simulink library "MESSIN_Library"  (R2024a)
settings: Solver=VariableStepAuto  StartTime=0.0  StopTime=10.0  RelTol=1e-3
undefined symbols (not defined in the file or in its folder): actuatorCommand, commandedActuator, commandMode, externCommand, ready, remoteControlDevice, sensor, supervisor, timestampUTC, useXNAllocation
libraries: $bdroot x376, etargetslib x52, simulink x19
(part 3 of 5)

== system MESSIN_Library/State Message/Pack MESSIN State Message/Pack INS ==
  insLFK100 : Inport
  Bus Selector : BusSelector  OutputSignals=timestampUTC,latitude,longitude,heave,velocityNorth,velocityEast,velocityDown,roll,pitch,heading,bodyAngularRateX,bodyAngularRateY,bodyAngularRateZ,bodyAccelerationX,bodyAccelerationY,bodyAccelerationZ,details.mode,details.systemFailure,details.reducedAccuracy,details.statusWord1,details.statusWord2
  Byte Pack5 : etargetslib/Byte Pack  datatypes={'double','double','double','double','double','double','double','double','double','double','double','double','double','double','double','double','uint8','uint8','uint16','uint16'}  byteAlign=1
  Convert Double Network Byte Order{1..4,6..7,9..11,15,17..22} (16 alike) : $bdroot/Utilities/Convert Double Network Byte Order
  Convert Uint16 Network Byte Order : $bdroot/Utilities/Convert Uint16 Network Byte Order
  Convert Uint16 Network Byte Order1 : $bdroot/Utilities/Convert Uint16 Network Byte Order
  Data Type Conversion{1..4,6..7,10,12..13,15..19,21,63} (16 alike) : DataTypeConversion  OutDataTypeStr=double  SaturateOnIntegerOverflow=off  RndMeth=Floor
  Data Type Conversion22 : DataTypeConversion  OutDataTypeStr=uint8  SaturateOnIntegerOverflow=off  RndMeth=Floor
  Data Type Conversion23 : DataTypeConversion  OutDataTypeStr=uint16  SaturateOnIntegerOverflow=off  RndMeth=Floor
  Data Type Conversion24 : DataTypeConversion  OutDataTypeStr=uint16  SaturateOnIntegerOverflow=off  RndMeth=Floor
  Subsystem : Subsystem
  bytes : Outport
  wires:
  insLFK100/1 -> Bus Selector/1
  Byte Pack5/1 -> bytes/1
  Data Type Conversion63/1 -> Convert Double Network Byte Order9/1
  Bus Selector/1 -> Data Type Conversion63/1  "<timestampUTC>"
  Bus Selector/2 -> Data Type Conversion1/1  "<latitude>"
  Bus Selector/3 -> Data Type Conversion3/1  "<longitude>"
  Bus Selector/4 -> Data Type Conversion2/1  "<heave>"
  Bus Selector/5 -> Data Type Conversion7/1  "<velocityNorth>"
  Bus Selector/6 -> Data Type Conversion4/1  "<velocityEast>"
  Bus Selector/7 -> Data Type Conversion6/1  "<velocityDown>"
  Bus Selector/10 -> Data Type Conversion12/1  "<heading>"
  Bus Selector/9 -> Data Type Conversion10/1  "<pitch>"
  Bus Selector/8 -> Data Type Conversion13/1  "<roll>"
  Data Type Conversion1/1 -> Convert Double Network Byte Order1/1
  Data Type Conversion3/1 -> Convert Double Network Byte Order3/1
  Data Type Conversion2/1 -> Convert Double Network Byte Order2/1
  Data Type Conversion7/1 -> Convert Double Network Byte Order7/1
  Data Type Conversion4/1 -> Convert Double Network Byte Order4/1
  Data Type Conversion6/1 -> Convert Double Network Byte Order6/1
  Data Type Conversion13/1 -> Convert Double Network Byte Order11/1
  Data Type Conversion10/1 -> Convert Double Network Byte Order10/1
  Data Type Conversion12/1 -> Convert Double Network Byte Order15/1
  Data Type Conversion18/1 -> Convert Double Network Byte Order20/1
  Data Type Conversion19/1 -> Convert Double Network Byte Order21/1
  Data Type Conversion17/1 -> Convert Double Network Byte Order19/1
  Data Type Conversion21/1 -> Convert Double Network Byte Order22/1
  Data Type Conversion15/1 -> Convert Double Network Byte Order17/1
  Data Type Conversion16/1 -> Convert Double Network Byte Order18/1
  Bus Selector/16 -> Data Type Conversion18/1  "<bodyAccelerationZ>"
  Bus Selector/15 -> Data Type Conversion19/1  "<bodyAccelerationY>"
  Bus Selector/14 -> Data Type Conversion17/1  "<bodyAccelerationX>"
  Bus Selector/13 -> Data Type Conversion21/1  "<bodyAngularRateZ>"
  Bus Selector/12 -> Data Type Conversion15/1  "<bodyAngularRateY>"
  Bus Selector/11 -> Data Type Conversion16/1  "<bodyAngularRateX>"
  Bus Selector/17 -> Data Type Conversion22/1  "<mode>"
  Bus Selector/20 -> Data Type Conversion23/1  "<statusWord1>"
  Bus Selector/21 -> Data Type Conversion24/1  "<statusWord2>"
  Data Type Conversion23/1 -> Convert Uint16 Network Byte Order/1
  Data Type Conversion24/1 -> Convert Uint16 Network Byte Order1/1
  Bus Selector/18 -> Subsystem/1(bit0)  "<systemFailure>"
  Bus Selector/19 -> Subsystem/2(bit1)  "<reducedAccuracy>"
  Convert Double Network Byte Order20/1 -> Byte Pack5/16
  Convert Double Network Byte Order21/1 -> Byte Pack5/15
  Convert Double Network Byte Order19/1 -> Byte Pack5/14
  Convert Double Network Byte Order22/1 -> Byte Pack5/13
  Convert Double Network Byte Order17/1 -> Byte Pack5/12
  Convert Double Network Byte Order18/1 -> Byte Pack5/11
  Convert Double Network Byte Order15/1 -> Byte Pack5/10
  Convert Double Network Byte Order10/1 -> Byte Pack5/9
  Convert Double Network Byte Order11/1 -> Byte Pack5/8
  Convert Double Network Byte Order6/1 -> Byte Pack5/7
  Convert Double Network Byte Order4/1 -> Byte Pack5/6
  Convert Double Network Byte Order7/1 -> Byte Pack5/5
  Convert Double Network Byte Order2/1 -> Byte Pack5/4
  Convert Double Network Byte Order3/1 -> Byte Pack5/3
  Convert Double Network Byte Order1/1 -> Byte Pack5/2
  Convert Double Network Byte Order9/1 -> Byte Pack5/1
  Data Type Conversion22/1 -> Byte Pack5/17
  Subsystem/1(byte) -> Byte Pack5/18
  Convert Uint16 Network Byte Order1/1 -> Byte Pack5/20
  Convert Uint16 Network Byte Order/1 -> Byte Pack5/19

== system MESSIN_Library/State Message/Pack MESSIN State Message/Pack Info ==
  messinState : Inport
  Bus Selector1 : BusSelector  OutputSignals=timestampUTC
  Byte Pack : etargetslib/Byte Pack  datatypes={'double'}  byteAlign=1
  Convert Double Network Byte Order : $bdroot/Utilities/Convert Double Network Byte Order
  bytes : Outport
  wires:
  Bus Selector1/1 -> Convert Double Network Byte Order/1  "<timestampUTC>"
  Convert Double Network Byte Order/1 -> Byte Pack/1
  messinState/1 -> Bus Selector1/1
  Byte Pack/1 -> bytes/1

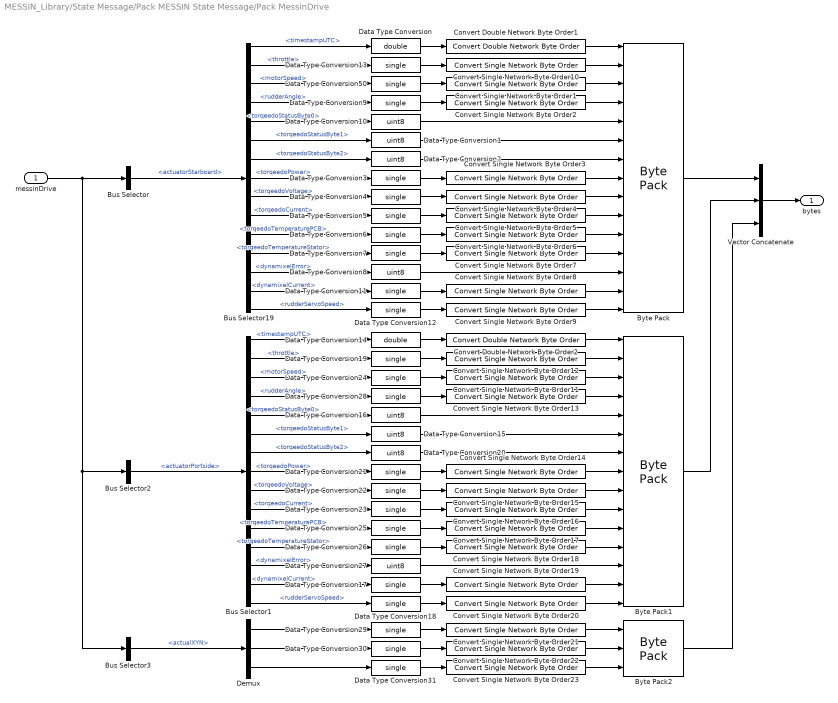
== system MESSIN_Library/State Message/Pack MESSIN State Message/Pack MessinDrive ==
  messinDrive : Inport
  Bus Selector : BusSelector  OutputSignals=actuatorStarboard
  Bus Selector1 : BusSelector  OutputSignals=timestampUTC,throttle,motorSpeed,rudderAngle,torqeedoStatusByte0,torqeedoStatusByte1,torqeedoStatusByte2,torqeedoPower,torqeedoVoltage,torqeedoCurrent,torqeedoTemperaturePCB,torqeedoTemperatureStator,dynamixelError,dynamixelCurrent,rudderServoSpeed
  Bus Selector19 : BusSelector  OutputSignals=timestampUTC,throttle,motorSpeed,rudderAngle,torqeedoStatusByte0,torqeedoStatusByte1,torqeedoStatusByte2,torqeedoPower,torqeedoVoltage,torqeedoCurrent,torqeedoTemperaturePCB,torqeedoTemperatureStator,dynamixelError,dynamixelCurrent,rudderServoSpeed
  Bus Selector2 : BusSelector  OutputSignals=actuatorPortside
  Bus Selector3 : BusSelector  OutputSignals=actualXYN
  Byte Pack : etargetslib/Byte Pack  datatypes={'double','single','single','single','uint8','uint8','uint8','single','single','single','single','single','uint8','single','single'}  byteAlign=1
  Byte Pack1 : etargetslib/Byte Pack  datatypes={'double','single','single','single','uint8','uint8','uint8','single','single','single','single','single','uint8','single','single'}  byteAlign=1
  Byte Pack2 : etargetslib/Byte Pack  datatypes={'single','single','single'}  byteAlign=1
  Convert Double Network Byte Order1 : $bdroot/Utilities/Convert Double Network Byte Order
  Convert Double Network Byte Order2 : $bdroot/Utilities/Convert Double Network Byte Order
  Convert Single Network Byte Order{1..23} (23 alike) : $bdroot/Utilities/Convert Single Network Byte Order
  Data Type Conversion : DataTypeConversion  OutDataTypeStr=double  SaturateOnIntegerOverflow=off  RndMeth=Floor
  Data Type Conversion{1..2,8,10,15..16,20,27} (8 alike) : DataTypeConversion  OutDataTypeStr=uint8  SaturateOnIntegerOverflow=off  RndMeth=Floor
  Data Type Conversion{3..7,9,11..13,17..19,21..26,28..31,50} (23 alike) : DataTypeConversion  OutDataTypeStr=single  SaturateOnIntegerOverflow=off  RndMeth=Floor
  Data Type Conversion14 : DataTypeConversion  OutDataTypeStr=double  SaturateOnIntegerOverflow=off  RndMeth=Floor
  Demux : Demux  Outputs=3
  Vector Concatenate : Concatenate  NumInputs=3
  bytes : Outport
  wires:
  Data Type Conversion/1 -> Convert Double Network Byte Order1/1
  Byte Pack/1 -> Vector Concatenate/1
  Vector Concatenate/1 -> bytes/1
  messinDrive/1 -> Bus Selector3/1, Bus Selector2/1, Bus Selector/1
  Bus Selector/1 -> Bus Selector19/1  "<actuatorStarboard>"
  Bus Selector19/1 -> Data Type Conversion/1  "<timestampUTC>"
  Bus Selector19/3 -> Data Type Conversion50/1  "<motorSpeed>"
  Data Type Conversion50/1 -> Convert Single Network Byte Order1/1
  Bus Selector19/4 -> Data Type Conversion9/1  "<rudderAngle>"
  Bus Selector19/5 -> Data Type Conversion10/1  "<torqeedoStatusByte0>"
  Data Type Conversion9/1 -> Convert Single Network Byte Order2/1
  Bus Selector19/6 -> Data Type Conversion1/1  "<torqeedoStatusByte1>"
  Bus Selector19/7 -> Data Type Conversion2/1  "<torqeedoStatusByte2>"
  Bus Selector19/8 -> Data Type Conversion3/1  "<torqeedoPower>"
  Bus Selector19/9 -> Data Type Conversion4/1  "<torqeedoVoltage>"
  Bus Selector19/10 -> Data Type Conversion5/1  "<torqeedoCurrent>"
  Bus Selector19/11 -> Data Type Conversion6/1  "<torqeedoTemperaturePCB>"
  Bus Selector19/12 -> Data Type Conversion7/1  "<torqeedoTemperatureStator>"
  Bus Selector19/13 -> Data Type Conversion8/1  "<dynamixelError>"
  Bus Selector19/14 -> Data Type Conversion11/1  "<dynamixelCurrent>"
  Bus Selector19/15 -> Data Type Conversion12/1  "<rudderServoSpeed>"
  Data Type Conversion3/1 -> Convert Single Network Byte Order3/1
  Data Type Conversion4/1 -> Convert Single Network Byte Order4/1
  Data Type Conversion5/1 -> Convert Single Network Byte Order5/1
  Data Type Conversion6/1 -> Convert Single Network Byte Order6/1
  Data Type Conversion7/1 -> Convert Single Network Byte Order7/1
  Data Type Conversion11/1 -> Convert Single Network Byte Order8/1
  Data Type Conversion12/1 -> Convert Single Network Byte Order9/1
  Data Type Conversion13/1 -> Convert Single Network Byte Order10/1
  Convert Double Network Byte Order1/1 -> Byte Pack/1
  Convert Single Network Byte Order10/1 -> Byte Pack/2
  Convert Single Network Byte Order1/1 -> Byte Pack/3
  Convert Single Network Byte Order2/1 -> Byte Pack/4
  Convert Single Network Byte Order3/1 -> Byte Pack/8
  Convert Single Network Byte Order4/1 -> Byte Pack/9
  Convert Single Network Byte Order5/1 -> Byte Pack/10
  Convert Single Network Byte Order6/1 -> Byte Pack/11
  Convert Single Network Byte Order7/1 -> Byte Pack/12
  Convert Single Network Byte Order8/1 -> Byte Pack/14
  Convert Single Network Byte Order9/1 -> Byte Pack/15
  Data Type Conversion10/1 -> Byte Pack/5
  Data Type Conversion1/1 -> Byte Pack/6
  Data Type Conversion2/1 -> Byte Pack/7
  Data Type Conversion8/1 -> Byte Pack/13
  Bus Selector19/2 -> Data Type Conversion13/1  "<throttle>"
  Bus Selector1/2 -> Data Type Conversion19/1  "<throttle>"
  Data Type Conversion27/1 -> Byte Pack1/13
  Data Type Conversion20/1 -> Byte Pack1/7
  Data Type Conversion15/1 -> Byte Pack1/6
  Data Type Conversion16/1 -> Byte Pack1/5
  Convert Single Network Byte Order20/1 -> Byte Pack1/15
  Convert Single Network Byte Order19/1 -> Byte Pack1/14
  Convert Single Network Byte Order18/1 -> Byte Pack1/12
  Convert Single Network Byte Order17/1 -> Byte Pack1/11
  Convert Single Network Byte Order16/1 -> Byte Pack1/10
  Convert Single Network Byte Order15/1 -> Byte Pack1/9
  Convert Single Network Byte Order14/1 -> Byte Pack1/8
  Convert Single Network Byte Order13/1 -> Byte Pack1/4
  Convert Single Network Byte Order11/1 -> Byte Pack1/3
  Convert Single Network Byte Order12/1 -> Byte Pack1/2
  Convert Double Network Byte Order2/1 -> Byte Pack1/1
  Data Type Conversion19/1 -> Convert Single Network Byte Order12/1
  Data Type Conversion18/1 -> Convert Single Network Byte Order20/1
  Data Type Conversion17/1 -> Convert Single Network Byte Order19/1
  Data Type Conversion26/1 -> Convert Single Network Byte Order18/1
  Data Type Conversion25/1 -> Convert Single Network Byte Order17/1
  Data Type Conversion23/1 -> Convert Single Network Byte Order16/1
  Data Type Conversion22/1 -> Convert Single Network Byte Order15/1
  Data Type Conversion21/1 -> Convert Single Network Byte Order14/1
  Bus Selector1/15 -> Data Type Conversion18/1  "<rudderServoSpeed>"
  Bus Selector1/14 -> Data Type Conversion17/1  "<dynamixelCurrent>"
  Bus Selector1/13 -> Data Type Conversion27/1  "<dynamixelError>"
  Bus Selector1/12 -> Data Type Conversion26/1  "<torqeedoTemperatureStator>"
  Bus Selector1/11 -> Data Type Conversion25/1  "<torqeedoTemperaturePCB>"
  Bus Selector1/10 -> Data Type Conversion23/1  "<torqeedoCurrent>"
  Bus Selector1/9 -> Data Type Conversion22/1  "<torqeedoVoltage>"
  Bus Selector1/8 -> Data Type Conversion21/1  "<torqeedoPower>"
  Bus Selector1/7 -> Data Type Conversion20/1  "<torqeedoStatusByte2>"
  Bus Selector1/6 -> Data Type Conversion15/1  "<torqeedoStatusByte1>"
  Data Type Conversion28/1 -> Convert Single Network Byte Order13/1
  Bus Selector1/5 -> Data Type Conversion16/1  "<torqeedoStatusByte0>"
  Bus Selector1/4 -> Data Type Conversion28/1  "<rudderAngle>"
  Data Type Conversion24/1 -> Convert Single Network Byte Order11/1
  Bus Selector1/3 -> Data Type Conversion24/1  "<motorSpeed>"
  Bus Selector1/1 -> Data Type Conversion14/1  "<timestampUTC>"
  Byte Pack1/1 -> Vector Concatenate/2
  Data Type Conversion14/1 -> Convert Double Network Byte Order2/1
  Bus Selector2/1 -> Bus Selector1/1  "<actuatorPortside>"
  Bus Selector3/1 -> Demux/1  "<actualXYN>"
  Demux/1 -> Data Type Conversion29/1
  Data Type Conversion29/1 -> Convert Single Network Byte Order21/1
  Data Type Conversion30/1 -> Convert Single Network Byte Order22/1
  Data Type Conversion31/1 -> Convert Single Network Byte Order23/1
  Demux/2 -> Data Type Conversion30/1
  Demux/3 -> Data Type Conversion31/1
  Convert Single Network Byte Order23/1 -> Byte Pack2/3
  Convert Single Network Byte Order22/1 -> Byte Pack2/2
  Convert Single Network Byte Order21/1 -> Byte Pack2/1
  Byte Pack2/1 -> Vector Concatenate/3

== system MESSIN_Library/State Message/Pack MESSIN State Message/Pack RCD ==
  rcd : Inport
  Bus Selector19 : BusSelector  OutputSignals=timestampUTC,joystickLeft,joystickRight
  Byte Pack : etargetslib/Byte Pack  datatypes={'double','single','single','single','single','single','single'}  byteAlign=1
  Convert Double Network Byte Order1 : $bdroot/Utilities/Convert Double Network Byte Order
  Convert Single Network Byte Order{1..6} (6 alike) : $bdroot/Utilities/Convert Single Network Byte Order
  Data Type Conversion : DataTypeConversion  OutDataTypeStr=double  SaturateOnIntegerOverflow=off  RndMeth=Floor
  Data Type Conversion{1..4,9,50} (6 alike) : DataTypeConversion  OutDataTypeStr=single  SaturateOnIntegerOverflow=off  RndMeth=Floor
  Demux : Demux  Outputs=3
  Demux1 : Demux  Outputs=3
  bytes : Outport
  wires:
  Data Type Conversion9/1 -> Convert Single Network Byte Order2/1
  Convert Single Network Byte Order2/1 -> Byte Pack/3
  Data Type Conversion50/1 -> Convert Single Network Byte Order1/1
  Bus Selector19/1 -> Data Type Conversion/1  "<timestampUTC>"
  rcd/1 -> Bus Selector19/1
  Convert Double Network Byte Order1/1 -> Byte Pack/1
  Data Type Conversion/1 -> Convert Double Network Byte Order1/1
  Convert Single Network Byte Order1/1 -> Byte Pack/2
  Byte Pack/1 -> bytes/1
  Data Type Conversion1/1 -> Convert Single Network Byte Order3/1
  Data Type Conversion2/1 -> Convert Single Network Byte Order6/1
  Data Type Conversion3/1 -> Convert Single Network Byte Order4/1
  Data Type Conversion4/1 -> Convert Single Network Byte Order5/1
  Demux/1 -> Data Type Conversion50/1
  Demux/2 -> Data Type Conversion9/1
  Demux/3 -> Data Type Conversion1/1
  Demux1/1 -> Data Type Conversion3/1
  Demux1/2 -> Data Type Conversion4/1
  Demux1/3 -> Data Type Conversion2/1
  Convert Single Network Byte Order3/1 -> Byte Pack/4
  Convert Single Network Byte Order4/1 -> Byte Pack/5
  Convert Single Network Byte Order5/1 -> Byte Pack/6
  Convert Single Network Byte Order6/1 -> Byte Pack/7
  Bus Selector19/2 -> Demux/1  "<joystickLeft>"
  Bus Selector19/3 -> Demux1/1  "<joystickRight>"

== system MESSIN_Library/State Message/Pack MESSIN State Message/Pack Supervisor ==
  supervisor : Inport
  Bus Selector1 : BusSelector  OutputSignals=internalOperationMode
  Bus Selector19 : BusSelector  OutputSignals=torqeedoPoweredOn,actuatorsEnabled,lightEnabled,actuatorsSynchronized,externModeEnabled
  Constant : Constant  Value=false  OutDataTypeStr=boolean
  Data Type Conversion : DataTypeConversion  OutDataTypeStr=uint8  SaturateOnIntegerOverflow=off  RndMeth=Floor
  Data Type Conversion1 : DataTypeConversion  OutDataTypeStr=uint8  SaturateOnIntegerOverflow=off  RndMeth=Floor
  Data Type Conversion2 : DataTypeConversion  OutDataTypeStr=boolean  SaturateOnIntegerOverflow=off  RndMeth=Floor
  Mux : Mux  Inputs=8
  Pack Bitfield : $bdroot/Utilities/Pack Bitfield
  Selector : Selector  InputPortWidth=8  IndexOptions=Index vector (dialog)  Indices=[8 7 6 5 4 3 2 1]  OutputSizes=1
  Vector Concatenate : Concatenate
  bytes : Outport
  wires:
  Vector Concatenate/1 -> bytes/1
  supervisor/1 -> Bus Selector1/1, Bus Selector19/1
  Bus Selector19/1 -> Mux/1  "<torqeedoPoweredOn>"
  Bus Selector19/2 -> Mux/2  "<actuatorsEnabled>"
  Bus Selector19/3 -> Mux/3  "<lightEnabled>"
  Bus Selector19/4 -> Mux/4  "<actuatorsSynchronized>"
  Bus Selector19/5 -> Mux/5  "<externModeEnabled>"
  Mux/1 -> Selector/1
  Constant/1 -> Mux/7, Mux/6, Mux/8
  Bus Selector1/1 -> Data Type Conversion1/1  "<internalOperationMode>"
  Pack Bitfield/1 -> Data Type Conversion/1
  Data Type Conversion/1 -> Vector Concatenate/1
  Data Type Conversion1/1 -> Vector Concatenate/2
  Selector/1 -> Data Type Conversion2/1
  Data Type Conversion2/1 -> Pack Bitfield/1

== system MESSIN_Library/State Message/Pack MESSIN State Message/Pack SystemDiagnostics ==
  systemDiagnostics : Inport
  Bus Selector1 : BusSelector  OutputSignals=details.hardware
  Bus Selector2 : BusSelector  OutputSignals=GNSS_OK,INS_OK,DVL_OK,ACTUATORS_OK,RCD_OK,EXTERN_OK
  Bus Selector3 : BusSelector  OutputSignals=details.network
  Bus Selector4 : BusSelector  OutputSignals=numTaskOverloads1,numTaskOverloads2,numTaskOverloads3,numCPUOverloads,numLostTicks,cpuTemperature
  Bus Selector5 : BusSelector  OutputSignals=internLinkUp,telemetryLinkUp,externLinkUp,internIncommingDataLFK100,internIncommingDataGNSSAsteRx3,internIncommingDataNortekDVL1000,internIncommingDataAirMAR,internIncommingDataBMS,internIncommingDataActuatorStarboard,internIncommingDataActuatorPortside,telemetryIncommingDataRCD,externIncommingData,firewallBlockedExternalInterface
  Bus Selector6 : BusSelector  OutputSignals=firewallAllowedExternalAddress
  Byte Pack : etargetslib/Byte Pack  datatypes={'uint32','uint32','uint32','uint32','uint32','single'}  byteAlign=1
  Byte Pack1 : etargetslib/Byte Pack  datatypes={'uint16','uint16','uint16','uint16','uint16'}  byteAlign=1
  Constant : Constant  Value=false  OutDataTypeStr=boolean
  Constant1 : Constant  Value=false  OutDataTypeStr=boolean
  Convert Single Network Byte Order : $bdroot/Utilities/Convert Single Network Byte Order
  Convert Uint16 Network Byte Order{,1..4} (5 alike) : $bdroot/Utilities/Convert Uint16 Network Byte Order
  Convert Uint32 Network Byte Order{,1..4} (5 alike) : $bdroot/Utilities/Convert Uint32 Network Byte Order
  Data Type Conversion{1..5} (5 alike) : DataTypeConversion  OutDataTypeStr=uint32  SaturateOnIntegerOverflow=off  RndMeth=Floor
  Data Type Conversion10 : DataTypeConversion  OutDataTypeStr=uint8  SaturateOnIntegerOverflow=off  RndMeth=Floor
  Data Type Conversion11 : DataTypeConversion  OutDataTypeStr=uint8  SaturateOnIntegerOverflow=off  RndMeth=Floor
  Data Type Conversion12 : DataTypeConversion  OutDataTypeStr=boolean  SaturateOnIntegerOverflow=off  RndMeth=Floor
  Data Type Conversion14 : DataTypeConversion  OutDataTypeStr=single  SaturateOnIntegerOverflow=off  RndMeth=Floor
  Data Type Conversion6 : DataTypeConversion  OutDataTypeStr=uint8  SaturateOnIntegerOverflow=off  RndMeth=Floor
  Data Type Conversion7 : DataTypeConversion  OutDataTypeStr=uint16  SaturateOnIntegerOverflow=off  RndMeth=Floor
  Data Type Conversion8 : DataTypeConversion  OutDataTypeStr=boolean  SaturateOnIntegerOverflow=off  RndMeth=Floor
  Data Type Conversion9 : DataTypeConversion  OutDataTypeStr=boolean  SaturateOnIntegerOverflow=off  RndMeth=Floor
  Demux : Demux  Outputs=5
  Mux : Mux  Inputs=8
  Mux1 : Mux  Inputs=8
  Mux2 : Mux  Inputs=8
  Pack Bitfield : $bdroot/Utilities/Pack Bitfield
  Pack Bitfield1 : $bdroot/Utilities/Pack Bitfield
  Pack Bitfield2 : $bdroot/Utilities/Pack Bitfield
  Selector : Selector  InputPortWidth=8  IndexOptions=Index vector (dialog)  Indices=[8 7 6 5 4 3 2 1]  OutputSizes=1
  Selector1 : Selector  InputPortWidth=8  IndexOptions=Index vector (dialog)  Indices=[8 7 6 5 4 3 2 1]  OutputSizes=1
  Selector2 : Selector  InputPortWidth=8  IndexOptions=Index vector (dialog)  Indices=[8 7 6 5 4 3 2 1]  OutputSizes=1
  Vector Concatenate : Concatenate  NumInputs=5
  bytes : Outport
  wires:
  systemDiagnostics/1 -> Bus Selector2/1, Bus Selector3/1, Bus Selector1/1
  Pack Bitfield/1 -> Data Type Conversion6/1
  Mux/1 -> Selector/1
  Constant/1 -> Mux/7, Mux/8
  Bus Selector1/1 -> Bus Selector4/1  "<hardware>"
  Bus Selector4/1 -> Data Type Conversion4/1  "<numTaskOverloads1>"
  Bus Selector4/2 -> Data Type Conversion1/1  "<numTaskOverloads2>"
  Bus Selector4/4 -> Data Type Conversion2/1  "<numCPUOverloads>"
  Bus Selector4/3 -> Data Type Conversion3/1  "<numTaskOverloads3>"
  Bus Selector4/5 -> Data Type Conversion5/1  "<numLostTicks>"
  Bus Selector3/1 -> Bus Selector6/1, Bus Selector5/1  "<network>"
  Constant1/1 -> Mux2/7, Mux2/6, Mux2/8
  Pack Bitfield1/1 -> Data Type Conversion10/1
  Mux1/1 -> Selector1/1
  Pack Bitfield2/1 -> Data Type Conversion11/1
  Mux2/1 -> Selector2/1
  Data Type Conversion4/1 -> Convert Uint32 Network Byte Order/1
  Data Type Conversion1/1 -> Convert Uint32 Network Byte Order1/1
  Data Type Conversion2/1 -> Convert Uint32 Network Byte Order3/1
  Data Type Conversion3/1 -> Convert Uint32 Network Byte Order2/1
  Data Type Conversion5/1 -> Convert Uint32 Network Byte Order4/1
  Byte Pack/1 -> Vector Concatenate/2
  Data Type Conversion6/1 -> Vector Concatenate/1
  Data Type Conversion10/1 -> Vector Concatenate/3
  Data Type Conversion11/1 -> Vector Concatenate/4
  Bus Selector6/1 -> Data Type Conversion7/1  "<firewallAllowedExternalAddress>"
  Data Type Conversion7/1 -> Demux/1
  Demux/1 -> Convert Uint16 Network Byte Order/1
  Demux/2 -> Convert Uint16 Network Byte Order1/1
  Demux/3 -> Convert Uint16 Network Byte Order2/1
  Demux/4 -> Convert Uint16 Network Byte Order3/1
  Demux/5 -> Convert Uint16 Network Byte Order4/1
  Byte Pack1/1 -> Vector Concatenate/5
  Vector Concatenate/1 -> bytes/1
  Selector/1 -> Data Type Conversion8/1
  Selector1/1 -> Data Type Conversion9/1
  Selector2/1 -> Data Type Conversion12/1
  Data Type Conversion8/1 -> Pack Bitfield/1
  Data Type Conversion9/1 -> Pack Bitfield1/1
  Data Type Conversion12/1 -> Pack Bitfield2/1
  Convert Uint16 Network Byte Order/1 -> Byte Pack1/1
  Convert Uint16 Network Byte Order1/1 -> Byte Pack1/2
  Convert Uint16 Network Byte Order2/1 -> Byte Pack1/3
  Convert Uint16 Network Byte Order3/1 -> Byte Pack1/4
  Convert Uint16 Network Byte Order4/1 -> Byte Pack1/5
  Bus Selector5/1 -> Mux1/1  "<internLinkUp>"
  Bus Selector5/2 -> Mux1/2  "<telemetryLinkUp>"
  Bus Selector5/3 -> Mux1/3  "<externLinkUp>"
  Bus Selector5/4 -> Mux1/4  "<internIncommingDataLFK100>"
  Bus Selector5/5 -> Mux1/5  "<internIncommingDataGNSSAsteRx3>"
  Bus Selector5/6 -> Mux1/6  "<internIncommingDataNortekDVL1000>"
  Bus Selector5/7 -> Mux1/7  "<internIncommingDataAirMAR>"
  Bus Selector5/8 -> Mux1/8  "<internIncommingDataBMS>"
  Bus Selector5/9 -> Mux2/1  "<internIncommingDataActuatorStarboard>"
  Bus Selector5/10 -> Mux2/2  "<internIncommingDataActuatorPortside>"
  Bus Selector5/11 -> Mux2/3  "<telemetryIncommingDataRCD>"
  Bus Selector5/12 -> Mux2/4  "<externIncommingData>"
  Bus Selector5/13 -> Mux2/5  "<firewallBlockedExternalInterface>"
  Bus Selector2/1 -> Mux/1  "<GNSS_OK>"
  Bus Selector2/2 -> Mux/2  "<INS_OK>"
  Bus Selector2/3 -> Mux/3  "<DVL_OK>"
  Bus Selector2/4 -> Mux/4  "<ACTUATORS_OK>"
  Bus Selector2/5 -> Mux/5  "<RCD_OK>"
  Bus Selector2/6 -> Mux/6  "<EXTERN_OK>"
  Data Type Conversion14/1 -> Convert Single Network Byte Order/1
  Bus Selector4/6 -> Data Type Conversion14/1  "<cpuTemperature>"
  Convert Single Network Byte Order/1 -> Byte Pack/6
  Convert Uint32 Network Byte Order4/1 -> Byte Pack/5
  Convert Uint32 Network Byte Order3/1 -> Byte Pack/4
  Convert Uint32 Network Byte Order2/1 -> Byte Pack/3
  Convert Uint32 Network Byte Order1/1 -> Byte Pack/2
  Convert Uint32 Network Byte Order/1 -> Byte Pack/1

== system MESSIN_Library/State Message/Unpack All MESSIN State Messages/run unpacking ==
  bytes : Inport
  length : Inport  Port=2
  numMessages : Inport  Port=3
  Enable : EnablePort
  Gain : Gain  Gain=0  OutDataTypeStr=uint32
  unpack all in a loop : Subsystem  TreatAsAtomicUnit=on
  messinState : Outport
  vecUnpacked : Outport  Port=2
  wires:
  bytes/1 -> unpack all in a loop/1(bytes)
  unpack all in a loop/1(messinState) -> messinState/1
  unpack all in a loop/2(vecUnpacked) -> vecUnpacked/1
  length/1 -> unpack all in a loop/2(length), Gain/1
  Gain/1 -> unpack all in a loop/4(zeros)
  numMessages/1 -> unpack all in a loop/3(numMessages)

== system MESSIN_Library/State Message/Unpack MESSIN State Message/is a valid message ==
  length : Inport
  bytes : Inport  Port=2
  AND1 : Logic  AllPortsSameDT=off  OutDataTypeStr=boolean
  CheckHeaderBytes : Subsystem  TreatAsAtomicUnit=on
  CheckMessageLength : simulink/Logic and Bit Operations/Compare To Constant  relop===  const=uint32(857)  OutDataTypeStr=boolean
  Min : MinMax  Inputs=2
  Width : Width  DataType=uint32
  validMessage : Outport
  wires:
  CheckMessageLength/1 -> AND1/1, CheckHeaderBytes/Enable
  AND1/1 -> validMessage/1
  CheckHeaderBytes/1(validHeader) -> AND1/2
  length/1 -> Min/1
  Width/1 -> Min/2
  bytes/1 -> CheckHeaderBytes/1(bytes), Width/1
  Min/1 -> CheckMessageLength/1

== system MESSIN_Library/State Message/Unpack MESSIN State Message/unpack message ==
  note: Sensor
  note: Info
  note: RCD
  note: Supervisor
  note: GNC
  note: SystemDiagnostics
  note: Extern Command
  bytes : Inport
  Enable : EnablePort
  Bytes 10 to 143 : Selector  IndexMode=Zero-based  IndexOptions=Index vector (dialog)  Indices=10:143  OutputSizes=1
  Bytes 144 to 193 : Selector  IndexMode=Zero-based  IndexOptions=Index vector (dialog)  Indices=144:193  OutputSizes=1
  Bytes 194 to 289 : Selector  IndexMode=Zero-based  IndexOptions=Index vector (dialog)  Indices=194:289  OutputSizes=1
  Bytes 2 to 9 : Selector  IndexMode=Zero-based  IndexOptions=Index vector (dialog)  Indices=2:9  OutputSizes=1
  Bytes 290 to 321 : Selector  IndexMode=Zero-based  IndexOptions=Index vector (dialog)  Indices=290:321  OutputSizes=1
  Bytes 322 to 369 : Selector  IndexMode=Zero-based  IndexOptions=Index vector (dialog)  Indices=322:369  OutputSizes=1
  Bytes 370 to 485 : Selector  IndexMode=Zero-based  IndexOptions=Index vector (dialog)  Indices=370:485  OutputSizes=1
  Bytes 486 to 517 : Selector  IndexMode=Zero-based  IndexOptions=Index vector (dialog)  Indices=486:517  OutputSizes=1
  Bytes 518 to 519 : Selector  IndexMode=Zero-based  IndexOptions=Index vector (dialog)  Indices=518:519  OutputSizes=1
  Bytes 520 to 721 : Selector  IndexMode=Zero-based  IndexOptions=Index vector (dialog)  Indices=520:721  OutputSizes=1
  Bytes 722 to 753 : Selector  IndexMode=Zero-based  IndexOptions=Index vector (dialog)  Indices=722:753  OutputSizes=1
  Bytes 754 to 790 : Selector  IndexMode=Zero-based  IndexOptions=Index vector (dialog)  Indices=754:790  OutputSizes=1
  Bytes 791 to 800 : Selector  IndexMode=Zero-based  IndexOptions=Index vector (dialog)  Indices=791:800  OutputSizes=1
  Bytes 801 to 832 : Selector  IndexMode=Zero-based  IndexOptions=Index vector (dialog)  Indices=801:832  OutputSizes=1
  Bytes 833 to 856 : Selector  IndexMode=Zero-based  IndexOptions=Index vector (dialog)  Indices=833:856  OutputSizes=1
  Empty MESSIN State Bus : $bdroot/State Message/Empty MESSIN State Bus
  Unpack ActuatorCommand : Subsystem
  Unpack AirMAR : Subsystem
  Unpack AllocationCommand : Subsystem
  Unpack BMS : Subsystem
  Unpack CommandedActuator : Subsystem
  Unpack DVL : Subsystem
  Unpack GNC : Subsystem
  Unpack GNSS : Subsystem
  Unpack INS : Subsystem
  Unpack Info : Subsystem
  Unpack Info1 : Subsystem
  Unpack MessinDrive : Subsystem
  Unpack RCD : Subsystem
  Unpack Supervisor : Subsystem
  Unpack SystemDiagnostics : Subsystem
  messinState : Outport
  wires:
  Unpack Info/1(busOut) -> Unpack INS/1(busIn)
  Bytes 2 to 9/1 -> Unpack Info/2(bytes)
  Empty MESSIN State Bus/1 -> Unpack Info/1(busIn)
  bytes/1 -> Bytes 2 to 9/1, Bytes 370 to 485/1, Bytes 791 to 800/1, Bytes 801 to 832/1, Bytes 833 to 856/1, Bytes 754 to 790/1, Bytes 722 to 753/1, Bytes 520 to 721/1, Bytes 518 to 519/1, Bytes 486 to 517/1, Bytes 322 to 369/1, Bytes 290 to 321/1, Bytes 194 to 289/1, Bytes 144 to 193/1, Bytes 10 to 143/1
  Unpack INS/1(busOut) -> Unpack GNSS/1(busIn)
  Unpack GNSS/1(busOut) -> Unpack DVL/1(busIn)
  Unpack DVL/1(busOut) -> Unpack AirMAR/1(busIn)
  Unpack AirMAR/1(busOut) -> Unpack BMS/1(busIn)
  Bytes 10 to 143/1 -> Unpack INS/2(bytes)
  Bytes 144 to 193/1 -> Unpack GNSS/2(bytes)
  Bytes 194 to 289/1 -> Unpack DVL/2(bytes)
  Bytes 290 to 321/1 -> Unpack AirMAR/2(bytes)
  Bytes 322 to 369/1 -> Unpack BMS/2(bytes)
  Unpack BMS/1(busOut) -> Unpack MessinDrive/1(busIn)
  Bytes 486 to 517/1 -> Unpack RCD/2(bytes)
  Unpack MessinDrive/1(busOut) -> Unpack RCD/1(busIn)
  Bytes 370 to 485/1 -> Unpack MessinDrive/2(bytes)
  Bytes 518 to 519/1 -> Unpack Supervisor/2(bytes)
  Unpack RCD/1(busOut) -> Unpack Supervisor/1(busIn)
  Unpack Supervisor/1(busOut) -> Unpack GNC/1(busIn)
  Bytes 520 to 721/1 -> Unpack GNC/2(bytes)
  Bytes 722 to 753/1 -> Unpack CommandedActuator/2(bytes)
  Unpack GNC/1(busOut) -> Unpack CommandedActuator/1(busIn)
  Bytes 754 to 790/1 -> Unpack SystemDiagnostics/2(bytes)
  Unpack CommandedActuator/1(busOut) -> Unpack SystemDiagnostics/1(busIn)
  Bytes 791 to 800/1 -> Unpack Info1/2(bytes)
  Unpack Info1/1(busOut) -> Unpack ActuatorCommand/1(busIn)
  Unpack ActuatorCommand/1(busOut) -> Unpack AllocationCommand/1(busIn)
  Unpack SystemDiagnostics/1(busOut) -> Unpack Info1/1(busIn)
  Unpack AllocationCommand/1(busOut) -> messinState/1
  Bytes 801 to 832/1 -> Unpack ActuatorCommand/2(bytes)
  Bytes 833 to 856/1 -> Unpack AllocationCommand/2(bytes)

== system MESSIN_Library/Command Message/Unpack All MESSIN Command Messages/run unpacking/unpack all in a loop ==
  bytes : Inport
  length : Inport  Port=2
  numMessages : Inport  Port=3
  zeros : Inport  Port=4
  Assignment : Assignment  DiagnosticForDimensions=Warning  IndexOptions=Index vector (port)  Indices=1  OutputSizes=1
  Data Type Conversion : DataTypeConversion  OutDataTypeStr=uint32  SaturateOnIntegerOverflow=off  RndMeth=Floor
  For Iterator : ForIterator  IterationSource=external  IterationVariableDataType=uint32
  Selector : Selector  IndexOptions=Index vector (port)  Indices=[1 3]  OutputSizes=1
  Selector2 : Selector  NumberOfDimensions=2  IndexOptions=Select all,Index vector (port)  Indices=[1 3],1  OutputSizes=1,1
  Unpack MESSIN Command Message : $bdroot/Command Message/Unpack MESSIN Command Message
  messinCommand : Outport
  vecUnpacked : Outport  Port=2
  wires:
  Data Type Conversion/1 -> Assignment/2
  For Iterator/1 -> Selector/2, Assignment/3, Selector2/2
  Assignment/1 -> vecUnpacked/1
  zeros/1 -> Assignment/1
  length/1 -> Selector/1
  bytes/1 -> Selector2/1
  numMessages/1 -> For Iterator/1
  Unpack MESSIN Command Message/1 -> Data Type Conversion/1
  Unpack MESSIN Command Message/2 -> messinCommand/1
  Selector2/1 -> Unpack MESSIN Command Message/1
  Selector/1 -> Unpack MESSIN Command Message/2

== system MESSIN_Library/Command Message/Unpack MESSIN Command Message/is a valid message/CheckHeaderBytes ==
  note: "MC"
  bytes : Inport
  Enable : EnablePort
  AND : Logic  AllPortsSameDT=off  OutDataTypeStr=boolean
  Compare To Constant : simulink/Logic and Bit Operations/Compare To Constant  relop===  const=uint8('M')  OutDataTypeStr=boolean
  Compare To Constant1 : simulink/Logic and Bit Operations/Compare To Constant  relop===  const=uint8('C')  OutDataTypeStr=boolean
  Demux : Demux  Outputs=2
  Selector : Selector  IndexOptions=Index vector (dialog)  Indices=1:2  OutputSizes=1
  validHeader : Outport
  wires:
  bytes/1 -> Selector/1
  Selector/1 -> Demux/1
  Demux/1 -> Compare To Constant/1
  Demux/2 -> Compare To Constant1/1
  Compare To Constant/1 -> AND/1
  Compare To Constant1/1 -> AND/2
  AND/1 -> validHeader/1

== system MESSIN_Library/Command Message/Unpack MESSIN Command Message/unpack message/Unpack ActuatorCommand ==
  busIn : Inport
  bytes : Inport  Port=2
  Bus Assignment : BusAssignment  AssignedSignals=actuatorCommand.throttleStarboard,actuatorCommand.throttlePortside,actuatorCommand.angleStarboard,actuatorCommand.anglePortside
  Byte Unpack : etargetslib/Byte Unpack  dimensions={1,1,1,1}  datatypes={'double','double','double','double'}  byteAlign=1
      settings: LibrarySourceBlock=embeddedtargetslib/Host Communication/Byte Unpack
  Convert Double Network Byte Order{,1..3} (4 alike) : $bdroot/Utilities/Convert Double Network Byte Order
  Make Finite{,1..3} (4 alike) : $bdroot/Utilities/Make Finite
  Signal Specification18 : SignalSpecification  OutDataTypeStr=double  Unit=1  Dimensions=1
  Signal Specification6 : SignalSpecification  OutDataTypeStr=double  Unit=1  Dimensions=1
  Signal Specification7 : SignalSpecification  OutDataTypeStr=double  Unit=rad  Dimensions=1
  Signal Specification8 : SignalSpecification  OutDataTypeStr=double  Unit=rad  Dimensions=1
  busOut : Outport
  wires:
  busIn/1 -> Bus Assignment/1
  bytes/1 -> Byte Unpack/1
  Bus Assignment/1 -> busOut/1
  Convert Double Network Byte Order/1 -> Make Finite/1
  Convert Double Network Byte Order1/1 -> Make Finite1/1
  Convert Double Network Byte Order2/1 -> Make Finite2/1
  Convert Double Network Byte Order3/1 -> Make Finite3/1
  Byte Unpack/1 -> Convert Double Network Byte Order/1
  Byte Unpack/2 -> Convert Double Network Byte Order1/1
  Byte Unpack/3 -> Convert Double Network Byte Order2/1
  Byte Unpack/4 -> Convert Double Network Byte Order3/1
  Make Finite/1 -> Signal Specification18/1
  Make Finite1/1 -> Signal Specification6/1
  Make Finite2/1 -> Signal Specification7/1
  Make Finite3/1 -> Signal Specification8/1
  Signal Specification18/1 -> Bus Assignment/2  "throttleStarboard"
  Signal Specification6/1 -> Bus Assignment/3  "throttlePortside"
  Signal Specification7/1 -> Bus Assignment/4  "angleStarboard"
  Signal Specification8/1 -> Bus Assignment/5  "anglePortside"

== system MESSIN_Library/Command Message/Unpack MESSIN Command Message/unpack message/Unpack AllocationCommand ==
  busIn : Inport
  bytes : Inport  Port=2
  Bus Assignment : BusAssignment  AssignedSignals=allocationCommand.XYN
  Byte Unpack : etargetslib/Byte Unpack  dimensions={1,1,1}  datatypes={'double','double','double'}  byteAlign=1
      settings: LibrarySourceBlock=embeddedtargetslib/Host Communication/Byte Unpack
  Convert Double Network Byte Order : $bdroot/Utilities/Convert Double Network Byte Order
  Convert Double Network Byte Order1 : $bdroot/Utilities/Convert Double Network Byte Order
  Convert Double Network Byte Order2 : $bdroot/Utilities/Convert Double Network Byte Order
  Make Finite : $bdroot/Utilities/Make Finite
  Make Finite1 : $bdroot/Utilities/Make Finite
  Make Finite2 : $bdroot/Utilities/Make Finite
  Mux : Mux  Inputs=3
  Signal Specification1 : SignalSpecification  OutDataTypeStr=double  Dimensions=3
  busOut : Outport
  wires:
  Byte Unpack/3 -> Convert Double Network Byte Order2/1
  Byte Unpack/2 -> Convert Double Network Byte Order1/1
  Byte Unpack/1 -> Convert Double Network Byte Order/1
  Convert Double Network Byte Order2/1 -> Make Finite2/1
  Convert Double Network Byte Order1/1 -> Make Finite1/1
  Convert Double Network Byte Order/1 -> Make Finite/1
  Bus Assignment/1 -> busOut/1
  bytes/1 -> Byte Unpack/1
  busIn/1 -> Bus Assignment/1
  Signal Specification1/1 -> Bus Assignment/2  "XYN"
  Make Finite2/1 -> Mux/3
  Make Finite1/1 -> Mux/2
  Make Finite/1 -> Mux/1
  Mux/1 -> Signal Specification1/1

== system MESSIN_Library/Command Message/Unpack MESSIN Command Message/unpack message/Unpack Info ==
  busIn : Inport
  bytes : Inport  Port=2
  Bus Assignment : BusAssignment  AssignedSignals=timestampUTC,ready,useXNAllocation,commandMode
  Byte Unpack : etargetslib/Byte Unpack  dimensions={1,1,1}  datatypes={'double','uint8','uint8'}  byteAlign=1
      settings: LibrarySourceBlock=embeddedtargetslib/Host Communication/Byte Unpack
  Convert Double Network Byte Order : $bdroot/Utilities/Convert Double Network Byte Order
  Data Type Conversion : DataTypeConversion  OutDataTypeStr=double  SaturateOnIntegerOverflow=off  RndMeth=Floor
  Data Type Conversion1 : DataTypeConversion  OutDataTypeStr=boolean  SaturateOnIntegerOverflow=off  RndMeth=Floor
  Make Finite : $bdroot/Utilities/Make Finite
  Selector : Selector  InputPortWidth=8  IndexOptions=Index vector (dialog)  Indices=8  OutputSizes=1
  Selector1 : Selector  InputPortWidth=8  IndexOptions=Index vector (dialog)  Indices=7  OutputSizes=1
  Signal Specification : SignalSpecification  OutDataTypeStr=double  Unit=s  Dimensions=1
  Signal Specification1 : SignalSpecification  OutDataTypeStr=boolean  Dimensions=1
  Signal Specification2 : SignalSpecification  OutDataTypeStr=boolean  Dimensions=1
  Unpack Bitfield : $bdroot/Utilities/Unpack Bitfield
  busOut : Outport
  wires:
  Bus Assignment/1 -> busOut/1
  bytes/1 -> Byte Unpack/1
  Byte Unpack/1 -> Convert Double Network Byte Order/1
  Convert Double Network Byte Order/1 -> Data Type Conversion/1
  busIn/1 -> Bus Assignment/1
  Signal Specification/1 -> Bus Assignment/2
  Data Type Conversion/1 -> Make Finite/1
  Make Finite/1 -> Signal Specification/1
  Byte Unpack/2 -> Unpack Bitfield/1
  Unpack Bitfield/1 -> Data Type Conversion1/1
  Data Type Conversion1/1 -> Selector1/1, Selector/1
  Selector/1 -> Signal Specification2/1
  Signal Specification2/1 -> Bus Assignment/3
  Byte Unpack/3 -> Bus Assignment/5
  Signal Specification1/1 -> Bus Assignment/4
  Selector1/1 -> Signal Specification1/1

== system MESSIN_Library/State Message/Pack MESSIN State Message/Pack ExternCommand/Pack ActuatorCommand ==
  actuatorCommand : Inport
  Bus Selector1 : BusSelector  OutputSignals=throttleStarboard,throttlePortside,angleStarboard,anglePortside
  Byte Pack : etargetslib/Byte Pack  datatypes={'double','double','double','double'}  byteAlign=1
  Convert Double Network Byte Order{,1..3} (4 alike) : $bdroot/Utilities/Convert Double Network Byte Order
  Data Type Conversion{,1..3} (4 alike) : DataTypeConversion  OutDataTypeStr=double  SaturateOnIntegerOverflow=off  RndMeth=Floor
  bytes : Outport
  wires:
  actuatorCommand/1 -> Bus Selector1/1
  Data Type Conversion3/1 -> Convert Double Network Byte Order3/1
  Data Type Conversion2/1 -> Convert Double Network Byte Order2/1
  Data Type Conversion1/1 -> Convert Double Network Byte Order1/1
  Data Type Conversion/1 -> Convert Double Network Byte Order/1
  Byte Pack/1 -> bytes/1
  Convert Double Network Byte Order/1 -> Byte Pack/1
  Convert Double Network Byte Order1/1 -> Byte Pack/2
  Convert Double Network Byte Order2/1 -> Byte Pack/3
  Convert Double Network Byte Order3/1 -> Byte Pack/4
  Bus Selector1/1 -> Data Type Conversion/1  "<throttleStarboard>"
  Bus Selector1/2 -> Data Type Conversion1/1  "<throttlePortside>"
  Bus Selector1/3 -> Data Type Conversion2/1  "<angleStarboard>"
  Bus Selector1/4 -> Data Type Conversion3/1  "<anglePortside>"

== system MESSIN_Library/State Message/Pack MESSIN State Message/Pack ExternCommand/Pack AllocationCommand ==
  allocationCommand : Inport
  Bus Selector1 : BusSelector  OutputSignals=XYN
  Byte Pack : etargetslib/Byte Pack  datatypes={'double','double','double'}  byteAlign=1
  Convert Double Network Byte Order : $bdroot/Utilities/Convert Double Network Byte Order
  Convert Double Network Byte Order1 : $bdroot/Utilities/Convert Double Network Byte Order
  Convert Double Network Byte Order2 : $bdroot/Utilities/Convert Double Network Byte Order
  Data Type Conversion : DataTypeConversion  OutDataTypeStr=double  SaturateOnIntegerOverflow=off  RndMeth=Floor
  Data Type Conversion1 : DataTypeConversion  OutDataTypeStr=double  SaturateOnIntegerOverflow=off  RndMeth=Floor
  Data Type Conversion2 : DataTypeConversion  OutDataTypeStr=double  SaturateOnIntegerOverflow=off  RndMeth=Floor
  Demux : Demux  Outputs=3
  bytes : Outport
  wires:
  Convert Double Network Byte Order2/1 -> Byte Pack/3
  Convert Double Network Byte Order1/1 -> Byte Pack/2
  Convert Double Network Byte Order/1 -> Byte Pack/1
  Byte Pack/1 -> bytes/1
  Data Type Conversion/1 -> Convert Double Network Byte Order/1
  Data Type Conversion1/1 -> Convert Double Network Byte Order1/1
  Data Type Conversion2/1 -> Convert Double Network Byte Order2/1
  allocationCommand/1 -> Bus Selector1/1
  Bus Selector1/1 -> Demux/1  "<XYN>"
  Demux/1 -> Data Type Conversion/1
  Demux/2 -> Data Type Conversion1/1
  Demux/3 -> Data Type Conversion2/1

== system MESSIN_Library/State Message/Pack MESSIN State Message/Pack ExternCommand/Pack Info ==
  externCommand : Inport
  Bus Selector1 : BusSelector  OutputSignals=timestampUTC
  Bus Selector2 : BusSelector  OutputSignals=ready,useXNAllocation
  Bus Selector3 : BusSelector  OutputSignals=commandMode
  Byte Pack : etargetslib/Byte Pack  datatypes={'double'}  byteAlign=1
  Cast To Boolean : DataTypeConversion  OutDataTypeStr=boolean  SaturateOnIntegerOverflow=off  RndMeth=Floor
  Cast To Boolean1 : DataTypeConversion  OutDataTypeStr=boolean  SaturateOnIntegerOverflow=off  RndMeth=Floor
  Constant : Constant  Value=false  OutDataTypeStr=boolean
  Convert Double Network Byte Order : $bdroot/Utilities/Convert Double Network Byte Order
  Data Type Conversion : DataTypeConversion  OutDataTypeStr=uint8  SaturateOnIntegerOverflow=off  RndMeth=Floor
  Mux : Mux  Inputs=8
  Pack Bitfield : $bdroot/Utilities/Pack Bitfield
  Selector : Selector  InputPortWidth=8  IndexOptions=Index vector (dialog)  Indices=[8 7 6 5 4 3 2 1]  OutputSizes=1
  Vector Concatenate : Concatenate  NumInputs=3
  bytes : Outport
  wires:
  Byte Pack/1 -> Vector Concatenate/1
  externCommand/1 -> Bus Selector3/1, Bus Selector2/1, Bus Selector1/1
  Convert Double Network Byte Order/1 -> Byte Pack/1
  Bus Selector1/1 -> Convert Double Network Byte Order/1  "<timestampUTC>"
  Cast To Boolean/1 -> Mux/1
  Constant/1 -> Mux/7, Mux/6, Mux/5, Mux/4, Mux/3, Mux/8
  Mux/1 -> Selector/1
  Selector/1 -> Pack Bitfield/1
  Bus Selector2/1 -> Cast To Boolean/1  "<ready>"
  Bus Selector3/1 -> Data Type Conversion/1  "<commandMode>"
  Pack Bitfield/1 -> Vector Concatenate/2
  Data Type Conversion/1 -> Vector Concatenate/3
  Vector Concatenate/1 -> bytes/1
  Cast To Boolean1/1 -> Mux/2
  Bus Selector2/2 -> Cast To Boolean1/1  "<useXNAllocation>"

== system MESSIN_Library/State Message/Pack MESSIN State Message/Pack INS/Subsystem ==
  bit0 : Inport
  bit1 : Inport  Port=2
  Constant : Constant  Value=false  OutDataTypeStr=boolean
  Data Type Conversion25 : DataTypeConversion  OutDataTypeStr=boolean  SaturateOnIntegerOverflow=off  RndMeth=Floor
  Data Type Conversion26 : DataTypeConversion  OutDataTypeStr=boolean  SaturateOnIntegerOverflow=off  RndMeth=Floor
  Mux : Mux  Inputs=8
  Pack Bitfield : $bdroot/Utilities/Pack Bitfield
  Selector : Selector  InputPortWidth=8  IndexOptions=Index vector (dialog)  Indices=[8 7 6 5 4 3 2 1]  OutputSizes=1
  byte : Outport
  wires:
  Constant/1 -> Mux/7, Mux/3, Mux/4, Mux/5, Mux/6, Mux/8
  Data Type Conversion26/1 -> Mux/2
  Pack Bitfield/1 -> byte/1
  Data Type Conversion25/1 -> Mux/1
  Mux/1 -> Selector/1
  bit1/1 -> Data Type Conversion26/1
  bit0/1 -> Data Type Conversion25/1
  Selector/1 -> Pack Bitfield/1

== system MESSIN_Library/State Message/Unpack All MESSIN State Messages/run unpacking/unpack all in a loop ==
  bytes : Inport
  length : Inport  Port=2
  numMessages : Inport  Port=3
  zeros : Inport  Port=4
  Assignment : Assignment  DiagnosticForDimensions=Warning  IndexOptions=Index vector (port)  Indices=1  OutputSizes=1
  Data Type Conversion : DataTypeConversion  OutDataTypeStr=uint32  SaturateOnIntegerOverflow=off  RndMeth=Floor
  For Iterator : ForIterator  IterationSource=external  IterationVariableDataType=uint32
  Selector : Selector  IndexOptions=Index vector (port)  Indices=[1 3]  OutputSizes=1
  Selector2 : Selector  NumberOfDimensions=2  IndexOptions=Select all,Index vector (port)  Indices=[1 3],1  OutputSizes=1,1
  Unpack MESSIN State Message : $bdroot/State Message/Unpack MESSIN State Message
  messinState : Outport
  vecUnpacked : Outport  Port=2
  wires:
  Data Type Conversion/1 -> Assignment/2
  For Iterator/1 -> Selector/2, Assignment/3, Selector2/2
  Assignment/1 -> vecUnpacked/1
  zeros/1 -> Assignment/1
  length/1 -> Selector/1
  bytes/1 -> Selector2/1
  numMessages/1 -> For Iterator/1
  Unpack MESSIN State Message/1 -> Data Type Conversion/1
  Unpack MESSIN State Message/2 -> messinState/1
  Selector2/1 -> Unpack MESSIN State Message/1
  Selector/1 -> Unpack MESSIN State Message/2

== system MESSIN_Library/State Message/Unpack MESSIN State Message/is a valid message/CheckHeaderBytes ==
  note: "MS"
  bytes : Inport
  Enable : EnablePort
  AND : Logic  AllPortsSameDT=off  OutDataTypeStr=boolean
  Compare To Constant : simulink/Logic and Bit Operations/Compare To Constant  relop===  const=uint8('M')  OutDataTypeStr=boolean
  Compare To Constant1 : simulink/Logic and Bit Operations/Compare To Constant  relop===  const=uint8('S')  OutDataTypeStr=boolean
  Demux : Demux  Outputs=2
  Selector : Selector  IndexOptions=Index vector (dialog)  Indices=1:2  OutputSizes=1
  validHeader : Outport
  wires:
  bytes/1 -> Selector/1
  Selector/1 -> Demux/1
  Demux/1 -> Compare To Constant/1
  Demux/2 -> Compare To Constant1/1
  Compare To Constant/1 -> AND/1
  Compare To Constant1/1 -> AND/2
  AND/1 -> validHeader/1

== system MESSIN_Library/State Message/Unpack MESSIN State Message/unpack message/Unpack ActuatorCommand ==
  busIn : Inport
  bytes : Inport  Port=2
  Bus Assignment : BusAssignment  AssignedSignals=externCommand.actuatorCommand.throttleStarboard,externCommand.actuatorCommand.throttlePortside,externCommand.actuatorCommand.angleStarboard,externCommand.actuatorCommand.anglePortside
  Byte Unpack : etargetslib/Byte Unpack  dimensions={1,1,1,1}  datatypes={'double','double','double','double'}  byteAlign=1
      settings: LibrarySourceBlock=embeddedtargetslib/Host Communication/Byte Unpack
  Convert Double Network Byte Order{,1..3} (4 alike) : $bdroot/Utilities/Convert Double Network Byte Order
  Make Finite{,1..3} (4 alike) : $bdroot/Utilities/Make Finite
  Signal Specification18 : SignalSpecification  OutDataTypeStr=double  Unit=1  Dimensions=1
  Signal Specification6 : SignalSpecification  OutDataTypeStr=double  Unit=1  Dimensions=1
  Signal Specification7 : SignalSpecification  OutDataTypeStr=double  Unit=rad  Dimensions=1
  Signal Specification8 : SignalSpecification  OutDataTypeStr=double  Unit=rad  Dimensions=1
  busOut : Outport
  wires:
  busIn/1 -> Bus Assignment/1
  bytes/1 -> Byte Unpack/1
  Bus Assignment/1 -> busOut/1
  Convert Double Network Byte Order/1 -> Make Finite/1
  Convert Double Network Byte Order1/1 -> Make Finite1/1
  Convert Double Network Byte Order2/1 -> Make Finite2/1
  Convert Double Network Byte Order3/1 -> Make Finite3/1
  Byte Unpack/1 -> Convert Double Network Byte Order/1
  Byte Unpack/2 -> Convert Double Network Byte Order1/1
  Byte Unpack/3 -> Convert Double Network Byte Order2/1
  Byte Unpack/4 -> Convert Double Network Byte Order3/1
  Make Finite/1 -> Signal Specification18/1
  Make Finite1/1 -> Signal Specification6/1
  Make Finite2/1 -> Signal Specification7/1
  Make Finite3/1 -> Signal Specification8/1
  Signal Specification18/1 -> Bus Assignment/2  "throttleStarboard"
  Signal Specification6/1 -> Bus Assignment/3  "throttlePortside"
  Signal Specification7/1 -> Bus Assignment/4  "angleStarboard"
  Signal Specification8/1 -> Bus Assignment/5  "anglePortside"
